simulink model "Model_Linearisierung_final"  (R2023b)
settings: Solver=FixedStepAuto  StartTime=0.0  StopTime=Inf  FixedStep=1e-4  RelTol=1e-3
PostLoadFcn:
  | if any(exist('dsrtsu_mdlpostloadfcn', 'file') ~= 0), dsrtsu_mdlpostloadfcn('Execute', bdroot); end
InitFcn:
  | , if any(exist('rtifpga_mdlclblib', 'file') ~= 0), rtifpga_mdlclblib('Init', bdroot); end,
  | , if any(exist('dsmpb_private', 'file') ~= 0), dsmpb_private('dsmpb_mdlclblib', 'Init', bdroot); end,
  | load('LUT_BRUSA_jax_grad.mat')
  | load('daten_nichtlinear_interpoliert.mat')
  | load('Maschinendaten.mat')
values from neighbouring files (symbols this model uses):
  delta_id = id_fine(2)-id_fine(1)    [Messdaten_Interpoliert.m]    (also in daten_nichtlinear_interpoliert.mat = 2.52525252525)
  delta_iq = iq_fine(2)-iq_fine(1)    [Messdaten_Interpoliert.m]    (also in daten_nichtlinear_interpoliert.mat = 5.05050505051)
  I_max = 170    [Maschinendaten.mat]    (also in Maschinendaten_Vorgabe.m; test_ModelParameters.m = evalin('base', 'I_max'); test_StrategySelection.m = tc.readConstant(tc.BLK_Imax))
  ID = [-250 -250 -250 -250 -250 -250 -250 -250 -250 -250 -250 -250 ... (10000 elements, 100x100)]    [daten_nichtlinear_interpoliert.mat]
  id_fine = linspace(min(id_vec), max(id_vec), 100)    [Messdaten_Interpoliert.m]    (also in daten_nichtlinear_interpoliert.mat = [-250 -247.474747475 -244.949494949 -242.424242424 -239.8989)
  IQ = [-250 -244.949494949 -239.898989899 -234.848484848 -229.797979798 -224.747474747 -219.696969697 -214.646464646 -209.595959596 -204.545454545 -199.494949495 -194.444444444 ... (10000 elements, 100x100)]    [daten_nichtlinear_interpoliert.mat]
  iq_fine = linspace(min(iq_vec), max(iq_vec), 100)    [Messdaten_Interpoliert.m]    (also in daten_nichtlinear_interpoliert.mat = [-250 -244.949494949 -239.898989899 -234.848484848 -229.7979)
  Ldd = Ldd_fine    [Messdaten_Interpoliert.m]    (also in daten_nichtlinear_interpoliert.mat = [0.000225276031415 0.000225750625371 0.000226241749969 0.000)
  Ldq = Ldq_fine    [Messdaten_Interpoliert.m]    (also in daten_nichtlinear_interpoliert.mat = [1.31113456519e-05 1.34236782585e-05 1.31001168558e-05 1.236)
  Lqd = Lqd_fine    [Messdaten_Interpoliert.m]    (also in daten_nichtlinear_interpoliert.mat = [7.22855329514e-05 7.00325573553e-05 6.7613098921e-05 6.5016)
  Lqq = Lqq_fine    [Messdaten_Interpoliert.m]    (also in daten_nichtlinear_interpoliert.mat = [0.000286039721686 0.000286453471045 0.000286025480511 0.000)
  n_max = 11000    [Maschinendaten.mat]    (also in Maschinendaten_Vorgabe.m; test_ModelParameters.m = evalin('base', 'n_max'); test_StrategySelection.m = tc.readConstant(tc.BLK_nmax))
  p = 3    [Maschinendaten.mat]    (also in Maschinendaten_Vorgabe.m; Messdaten_Interpoliert.m; test_ModelParameters.m = evalin('base', 'p'))
  Psid = Psid_fine    [Messdaten_Interpoliert.m]    (also in daten_nichtlinear_interpoliert.mat = [0.00602681114795 0.00609490588107 0.00615917040906 0.006219)
  Psiq = Psiq_fine    [Messdaten_Interpoliert.m]    (also in daten_nichtlinear_interpoliert.mat = [-0.166252688687 -0.164805403122 -0.163363500753 -0.16192610)
  Rs = 0.018    [Maschinendaten.mat]    (also in Maschinendaten_Vorgabe.m; test_ModelParameters.m = evalin('base', 'Rs'))
  U_dc = 560    [Maschinendaten.mat]    (also in Maschinendaten_Vorgabe.m; test_ModelParameters.m = evalin('base', 'U_dc'))
  U_max = 323.316150746    [Maschinendaten.mat]    (also in Maschinendaten_Vorgabe.m = U_dc / sqrt(3); test_ModelParameters.m = evalin('base', 'U_max'))
(part 3 of 3)

== matlab function Model_Linearisierung_final/Subsystem Arbeitspunktsteuerung/Arbeitspunktsteuerung/Linearisierung um idq0 ==
  data: start_cmd input; id_init input; id0_out output; iq_init input; id_iter input; iq_iter input; id_fine input; iq_fine input; Psid input; Psiq input; Schrittweite_id input; Schrittweite_iq input; delta_id_last input; delta_iq_last input; iq0_out output; L_dd0 output; L_qq0 output; L_dq0 output; L_qd0 output; psid_d output; psiq_q output; psi_d0 output; psi_q0 output; psi_bar_d output; psi_bar_q output
function [id0_out, iq0_out, L_dd0, L_qq0, L_dq0, L_qd0, ...
          psid_d, psiq_q, psi_d0, psi_q0, psi_bar_d, psi_bar_q] = ...
    fcn(start_cmd, id_init, iq_init, id_iter, iq_iter, ...
        id_fine, iq_fine, Psid, Psiq, Schrittweite_id, Schrittweite_iq, delta_id_last, delta_iq_last)
%#codegen
%
% BLOCK 1: Lokale Linearisierung der LUT-Flüsse
%
% Ziel:
%   Bestimmung der lokalen Induktivitäten um den aktuellen Arbeitspunkt
%
%   psi_d ~= psi_d0 + L_dd*(id-id0) + L_dq*(iq-iq0)
%   psi_q ~= psi_q0 + L_qd*(id-id0) + L_qq*(iq-iq0)
%   ψd ~= ψd0 ​+ Ldd​*(id​−id0​) + Ldq​*(iq​−iq0​)

% Für die Hackl-Berechnung wird anschließend eine gemeinsame
% Kreuzinduktivität verwendet
%   L_m = (L_dq + L_qd)/2

%% ============================================================
% 1. Feste Permanentmagnetflussanteile
% =============================================================
psi_pm_d0 = 0.0718; % Permanentmagnetfluss

% Initialisierung
psi_d0 = psi_pm_d0;
psi_q0 = 0.0;
psid_d = 0.0;    % Fluss Psid = psid0 + L_diff*delta_I
psiq_q = 0.0;
psi_bar_d = 0.0;
psi_bar_q = 0.0;

%% ============================================================
% 2. Grenzen der LUT bestimmen
% =============================================================
id_min = id_fine(1);
id_max = id_fine(end);

iq_min = iq_fine(1);
iq_max = iq_fine(end);

%% ============================================================
% 3. Wahl des aktuellen Arbeitspunktes
% =============================================================
if start_cmd
    % Erster geschätzter Arbeitspunkt
    id0  = id_init;
    iq0  = iq_init;
    delta_ID    = 0.0;
    delta_IQ    = 0.0;
else
    % Arbeitspunkt und delta I aus vorheriger Iteration
    id0 = id_iter;
    iq0 = iq_iter;
    delta_ID = delta_id_last;
    delta_IQ = delta_iq_last;
end

%% ============================================================
% 4. Arbeitspunkt auf LUT-Bereich begrenzen
% =============================================================
id0 = min(max(id0, id_min), id_max);
iq0 = min(max(iq0, iq_min), iq_max);

%% ============================================================
% 5. Gültigkeitsprüfung der Differenzschritte
% =============================================================
valid = true;

if ~isfinite(Schrittweite_id) || ~isfinite(Schrittweite_iq) || ...
   Schrittweite_id <= 0 || Schrittweite_iq <= 0

    valid = false;

    id0_out = id0;
    iq0_out = iq0;

    L_dd0 = 0;
    L_qq0 = 0;
    L_dq0 = 0;
    L_qd0 = 0;
    L_m0  = 0;

    return;
end

%% ============================================================
% 6. Gesamtflüsse am Arbeitspunkt bestimmen: ψd0(id0,iq0)​
% =============================================================
psi_d0 = interp2(id_fine, iq_fine, Psid, id0, iq0, 'linear');

psi_q0 = interp2(id_fine, iq_fine, Psiq, id0, iq0, 'linear');

%% ============================================================
% 7. Tatsächliche Differenzschritte bestimmen
% =============================================================
% Schritt darf nicht über die LUT-Grenze hinausgehen.
h_d_minus = min(Schrittweite_id, id0 - id_min);
h_d_plus  = min(Schrittweite_id, id_max - id0);

h_q_minus = min(Schrittweite_iq, iq0 - iq_min);
h_q_plus  = min(Schrittweite_iq, iq_max - iq0);


%% ============================================================
% 8. L_dd = d psi_d / d id
% =============================================================
if h_d_minus > 0 && h_d_plus > 0

    % Zentrale Differenz
    psi_d_plus = interp2(id_fine, iq_fine, Psid, ...
                         id0 + h_d_plus, iq0, 'linear');

    psi_d_minus = interp2(id_fine, iq_fine, Psid, ...
                          id0 - h_d_minus, iq0, 'linear');

    L_dd0 = (psi_d_plus - psi_d_minus) / ...
            (h_d_plus + h_d_minus);

elseif h_d_plus > 0

    % Vorwärtsdifferenz
    psi_d_plus = interp2(id_fine, iq_fine, Psid, ...
                         id0 + h_d_plus, iq0, 'linear');

    L_dd0 = (psi_d_plus - psi_d0) / h_d_plus;

elseif h_d_minus > 0

    % Rückwärtsdifferenz
    psi_d_minus = interp2(id_fine, iq_fine, Psid, ...
                          id0 - h_d_minus, iq0, 'linear');

    L_dd0 = (psi_d0 - psi_d_minus) / h_d_minus;

else

    L_dd0 = NaN;

end


%% ============================================================
% 9. L_dq = d psi_d / d iq
% =============================================================

if h_q_minus > 0 && h_q_plus > 0

    % Zentrale Differenz
    psi_d_plus_q = interp2(id_fine, iq_fine, Psid, ...
                           id0, iq0 + h_q_plus, 'linear');

    psi_d_minus_q = interp2(id_fine, iq_fine, Psid, ...
                            id0, iq0 - h_q_minus, 'linear');

    L_dq0 = (psi_d_plus_q - psi_d_minus_q) / ...
            (h_q_plus + h_q_minus);

elseif h_q_plus > 0

    % Vorwärtsdifferenz
    psi_d_plus_q = interp2(id_fine, iq_fine, Psid, ...
                           id0, iq0 + h_q_plus, 'linear');

    L_dq0 = (psi_d_plus_q - psi_d0) / h_q_plus;

elseif h_q_minus > 0

    % Rückwärtsdifferenz
    psi_d_minus_q = interp2(id_fine, iq_fine, Psid, ...
                            id0, iq0 - h_q_minus, 'linear');

    L_dq0 = (psi_d0 - psi_d_minus_q) / h_q_minus;

else

    L_dq0 = NaN;

end


%% ============================================================
% 10. L_qd = d psi_q / d id
% =============================================================

if h_d_minus > 0 && h_d_plus > 0

    % Zentrale Differenz
    psi_q_plus_d = interp2(id_fine, iq_fine, Psiq, ...
                           id0 + h_d_plus, iq0, 'linear');

    psi_q_minus_d = interp2(id_fine, iq_fine, Psiq, ...
                            id0 - h_d_minus, iq0, 'linear');

    L_qd0 = (psi_q_plus_d - psi_q_minus_d) / ...
            (h_d_plus + h_d_minus);

elseif h_d_plus > 0

    % Vorwärtsdifferenz
    psi_q_plus_d = interp2(id_fine, iq_fine, Psiq, ...
                           id0 + h_d_plus, iq0, 'linear');

    L_qd0 = (psi_q_plus_d - psi_q0) / h_d_plus;

elseif h_d_minus > 0

    % Rückwärtsdifferenz
    psi_q_minus_d = interp2(id_fine, iq_fine, Psiq, ...
                            id0 - h_d_minus, iq0, 'linear');

    L_qd0 = (psi_q0 - psi_q_minus_d) / h_d_minus;

else

    L_qd0 = NaN;

end


%% ============================================================
% 11. L_qq = d psi_q / d iq
% =============================================================
if h_q_minus > 0 && h_q_plus > 0

    % Zentrale Differenz
    psi_q_plus_q = interp2(id_fine, iq_fine, Psiq, ...
                           id0, iq0 + h_q_plus, 'linear');

    psi_q_minus_q = interp2(id_fine, iq_fine, Psiq, ...
                            id0, iq0 - h_q_minus, 'linear');

    L_qq0 = (psi_q_plus_q - psi_q_minus_q) / ...
            (h_q_plus + h_q_minus) ;

elseif h_q_plus > 0

    % Vorwärtsdifferenz
    psi_q_plus_q = interp2(id_fine, iq_fine, Psiq, ...
                           id0, iq0 + h_q_plus, 'linear');

    L_qq0 = (psi_q_plus_q - psi_q0) / h_q_plus ;

elseif h_q_minus > 0

    % Rückwärtsdifferenz
    psi_q_minus_q = interp2(id_fine, iq_fine, Psiq, ...
                            id0, iq0 - h_q_minus, 'linear');

    L_qq0 = (psi_q0 - psi_q_minus_q) / h_q_minus ;

else

    L_qq0 = NaN;

end


%% ============================================================
% 12. Kreuzkopplung auf eine gemeinsame lokale Induktivität
% =============================================================
% lokale Jacobi-Matrix der Flüsse:        Hackl: 
%       [ L_dd   L_dq ]             L_m = (L_dq + L_qd)/2
%   L = [             ]
%       [ L_qd   L_qq ]
if isfinite(L_dq0) && isfinite(L_qd0)
    L_m0 = 0.5 * (L_dq0 + L_qd0);
else
    L_m0 = NaN;
end

%% ============================================================
% 13. Konsistenzprüfung (alle Werte endlich?)
% =============================================================
if ~isfinite(psi_d0) || ~isfinite(psi_q0) || ...
   ~isfinite(L_dd0) || ~isfinite(L_qq0) || ...
   ~isfinite(L_dq0) || ~isfinite(L_qd0) || ...
   ~isfinite(L_m0)

    valid = false;
end

% Gesamtflüsse: ψd ​= ψd0 ​+ Ldd*​(id​−id0​) + Ldq*​(iq​−iq0​)
psid_d = psi_d0 + L_dd0*delta_ID + L_dq0*delta_IQ;
psiq_q = psi_q0 + L_qd0*delta_ID + L_qq0*delta_IQ;

% Offset lokaler linearer Fluss (Konstantanteil pro Iteration)
% ψd_quer ​= ψd0 ​- Ldd*​id0​ - Ldq*​iq0​
psi_bar_d = psi_d0 - L_dd0*id0 - L_dq0*iq0;
psi_bar_q = psi_q0 - L_qd0*id0 - L_qq0*iq0;

%% ============================================================
% 14. Ausgangsarbeitspunkt
% =============================================================
id0_out = id0;
iq0_out = iq0;

end

== matlab function Model_Linearisierung_final/Subsystem Arbeitspunktsteuerung/Arbeitspunktsteuerung/Quadriken Hackl ==
  data: Ldd input; Lqq input; Ldq input; Lqd input; omega input; p input; Rs input; psi_bar_d input; psi_bar_q input; Imax input; Umax input; q_current output size=[1 6]; q_voltage output size=[1 6]; T_soll input; q_torque output size=[1 6]; q_MTPC output size=[1 6]; q_MTPV output size=[1 6]
function [q_current, q_voltage, q_torque, q_MTPC, q_MTPV] = ...
    Quadriken (Ldd, Lqq, Ldq, Lqd, omega, p, Rs, psi_bar_d, psi_bar_q, ...
               Imax, Umax, T_soll)
% Variablen
psi_pm_d = 0.0718; % Permanentmagnetfluss
psi_pm_q = 0.0;
Lm = 0.5* (Ldq + Lqd);
K = 1.5*p;

% Allgemeine Form:
% F(id,iq) = a*id^2 + b*id*iq + c*iq^2 + d*id + e*iq+ f
% q = [a b c d e f]
% --------------------------------------------------------------
%% 1. Stromkreis
% Allgemein: F(id,iq) = a*id^2 + b*id*iq + c*iq^2 + d*id + e*iq+ f
% Strom: id^2 + iq^2 - Imax^2 = 0
q_current = [ 1, 0, 1, 0, 0, -Imax^2 ];

%% 2. Spannungsellipse
a = (Rs - omega*Lqd)^2 + (omega*Ldd)^2;

b = 2*((Rs - omega*Lqd)*(-omega*Lqq)+ (omega*Ldd)*(Rs + omega*Ldq));

c = (omega*Lqq)^2 + (Rs + omega*Ldq)^2;

d = 2*((Rs - omega*Lqd)*(-omega*psi_bar_q) + (omega*Ldd)*(omega*psi_bar_d));

e = 2*((-omega*Lqq)*(-omega*psi_bar_q) + (Rs + omega*Ldq)*(omega*psi_bar_d));

f = omega^2*(psi_bar_d^2 + psi_bar_q^2) - Umax^2;

q_voltage = [a b c d e f];

%% 3. Drehmomentkennlinie
% T = K * [Psid*Iq - Psiq*Id]
% T - T_soll = 0
% => q_torque
% Hackl
q_torque = [-K*Lqd, K*(Ldd-Lqq), K*Ldq, -K*psi_bar_q, K*psi_bar_d, -T_soll ];

%% 4. MTPC
% lokal konstanter Flussanteil psi_bar_d/q
% -> beschreibt lokal linearisiertes Flussmodell
% Mc11*id^2 + 2*Mc12*id*iq + Mc22*iq^2 + 2*mc1*id + 2*mc2*iq = 0
Mc11 = K*(Ldd-Lqq)/2;
Mc12 = K*Lm;
Mc22 = -K*(Ldd-Lqq)/2;

mc1 = K*psi_bar_d/4;
mc2 = K*psi_bar_q/4;

q_MTPC = [ Mc11, 2*Mc12, Mc22, 2*mc1, 2*mc2, 0 ];

%% 5. MTPV 
% lokal konstanter Flussanteil psi_bar_d/q 
% Mv11*id^2 + 2*Mv12*id*iq + Mv22*iq^2 + 2*mv1*id + 2*mv2*iq + mu_v = 0
Mv11 = K*(omega^2*Lm^2*(Ldd+Lqq) + (Ldd-Lqq)/2 * ...
      (Rs^2 + omega^2*(Ldd^2+Lm^2)) );

Mv12 = K*(Lm/2 * (2*Rs^2 + omega^2*(Ldd^2+Lqq^2+2*Lm^2)) );

Mv22 = K*(omega^2*Lm^2*(Ldd+Lqq) - (Ldd-Lqq)/2 * ...
      (Rs^2 + omega^2*(Lqq^2+Lm^2)) );

mv1 = K*((Rs^2 + omega^2*(2*Ldd^2-Ldd*Lqq+3*Lm^2)) *psi_bar_d/4 ...
    + omega^2*Lm*(Ldd+Lqq)*psi_bar_q/2 );

mv2 = K*(omega^2*Lm*(Ldd+Lqq)*psi_bar_d/2 ...
    + (Rs^2 + omega^2*(2*Ldd^2-Ldd*Lqq+3*Lm^2)) *psi_bar_q/4 );

mu_v = 0.75*p*omega^2*(Ldd*psi_bar_d^2 ...
    + 2*Lm*psi_bar_d*psi_bar_q + Lqq*psi_bar_q^2 );

q_MTPV = [Mv11, 2*Mv12, Mv22, 2*mv1, 2*mv2, mu_v ];

%% 5. MTPF 
% % wird in Glac nicht verwendet
% Mf11 = 1.5*p*((Ldd-Lqq)/2 *(Ldd^2+Lm^2) + Lm^2 *(Ldd+Lqq) );
% Mf12 = 1.5*p*(Lm/2 *(Ldd^2+Lqq^2+2*Lm^2) );
% Mf22 = 1.5*p*( -(Ldd-Lqq)/2 *(Lqq^2+Lm^2) + Lm^2*(Ldd+Lqq) );
% 
% mf1 = 1.5*p*((2*Ldd^2 - Ldd*Lqq + 3*Lm^2)*psi_pm_d/4 ...
%     + Lm*(Ldd+Lqq)*psi_pm_q/2 );
% mf2 = 1.5*p*(Lm*(Ldd+Lqq)*psi_pm_d/2 + (2*Lqq^2-Ldd*Lqq+3*Lm^2)*psi_pm_q/4);
% 
% mu_f = 0.75*p*(Ldd*psi_pm_d^2 + 2*Lm*psi_pm_d*psi_pm_q + Lqq*psi_pm_q^2 );
% 
% f_MTPF = Mf11*ID.^2 + 2*Mf12*ID.*IQ + Mf22*IQ.^2 + 2*(mf1.*ID + mf2.*IQ) + mu_f;
